simulink model "part1"  (R2020a)
settings: Solver=VariableStepAuto  StartTime=0.0  StopTime=1000  RelTol=1e-3
values from neighbouring files (symbols this model uses):
  beta_c_init = 30    [init.m]    (also in simulation1.m = 2.35619449019; simulation2.m = 3.14159265359; simulation3.m = 0; simulation4.m = 0)
  beta_c_slope = 90/1000    (= 0.09)    [init.m]    (also in simulation1.m = 0; simulation2.m = 0.00235619449019; simulation3.m = 0; simulation4.m = 0)
  eta_d = [50 0 0; 50 -50 0; 50 -50 pi/2; 0 -50 pi/2; 0 0 0]    [init.m]    (also in simulation1.m = [0 0 0; 0 0 0]; simulation2.m = [0 0 0; 0 0 0]; simulation3.m = [0 0 0; 10 10 3*pi/2]; simulation4.m = [0 0 0; 50 0 0; 50 -50 0; 50 -50 -pi/4; 0 -50 -pi/4; 0 0 0])
  Kd = eye(n)*kd    [control_law.m]
  Ki = eye(n)*ki    [control_law.m]    (also in lqr_error.m = lqr(Aa,Ba,Qa,R); lqr_integral.m = lqr(Aa,Ba,Qa,R))
  Kp = eye(n)*kp    [control_law.m]
  V_c = input    [gui.m]    (also in init.m = 0.5; simulation1.m = 0.5; simulation2.m = 0.5; simulation3.m = 0)
undefined symbols (not defined in the file or in its folder): DiscIntNeverNeededParam, Hoerner, vessel
libraries: marine_gnc x11, simulink x2, marine_hydro x1
settings Model: OrderedModelArguments=off  Creator=jonbjor  LastModifiedBy=magnushaukeland
settings DataIOCC: ReturnWorkspaceOutputs=off
settings DebuggingCC: ArithmeticOperatorsInVariantConditions=warning
settings SFSimCC: SimUseLocalCustomCode=off  CustomCodeUndefinedFunction=UseInterfaceOnly
settings RTWCC: RTWUseLocalCustomCode=off

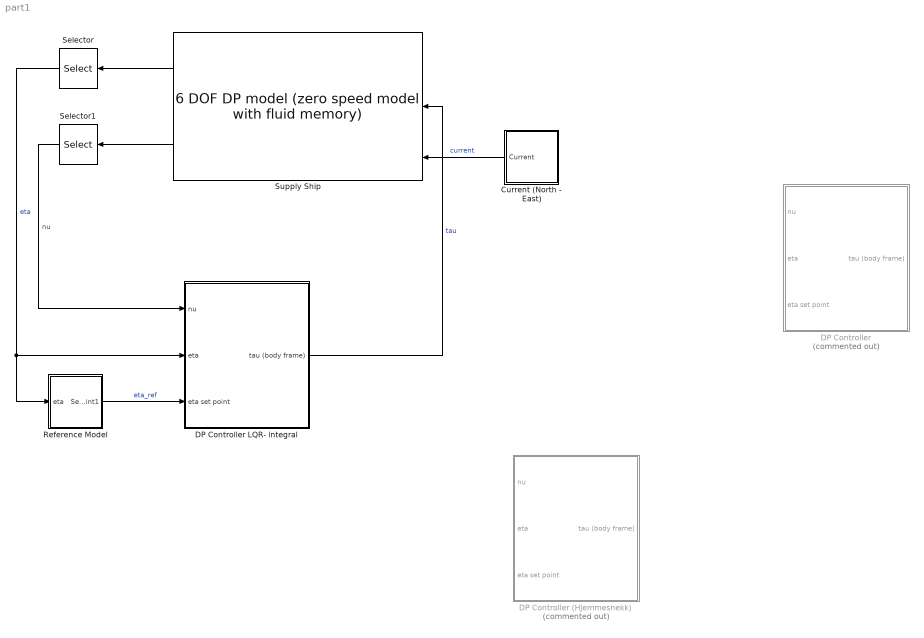
== system part1 ==
  Current (North - East) : Subsystem
  DP Controller : Subsystem  Commented=on
  DP Controller (Hjemmesnekk) : Subsystem  Commented=on
  DP Controller LQR- integral : Subsystem
  Reference Model : Subsystem
  Selector : Selector  InputPortWidth=6  IndexOptions=Index vector (dialog)  Indices=[1 2 6]  OutputSizes=1
  Selector1 : Selector  InputPortWidth=6  IndexOptions=Index vector (dialog)  Indices=[1 2 6]  OutputSizes=1
  Supply Ship : marine_hydro/Hydro Library/6 DOF DP model  (zero speed model with fluid memory)  ABC=vesselABC  rho=1025  Axc=0.9*vessel.main.T*vessel.main.B  Ayc=0.9*vessel.main.T*vessel.main.Lpp  CX=1  CY_2D=Hoerner(vessel.main.B,vessel.main.T)  Bv=vessel.Bv  mask(6 DOF zero speed model){}
      link override "Integrator1 ": InitialCondition=nu0
      link override Integrator2: InitialCondition=eta0
      settings: SourceProductName=MSS Hydro
      mask Display:
      | image('supply.jpg');
      | color('white'); port_label('output', 1, 'eta')
      | color('white'); port_label('output', 2, 'nu')
      | color('white'); port_label('input', 1, 'tau_wave')
      | color('white'); port_label('input', 2, 'tau')
      | color('white'); port_label('input', 3, 'nu_c')
  wires:
  Current (North - East)/1(Current) -> Supply Ship/3  "current"
  Supply Ship/1 -> Selector/1
  Supply Ship/2 -> Selector1/1
  Selector/1 -> DP Controller LQR- integral/2(eta), Reference Model/1(eta)  "eta"
  Reference Model/1(Set-point1) -> DP Controller LQR- integral/3(eta set point)  "eta_ref"
  Selector1/1 -> DP Controller LQR- integral/1(nu)  "nu"
  DP Controller LQR- integral/1(tau (body frame)) -> Supply Ship/2  "tau"

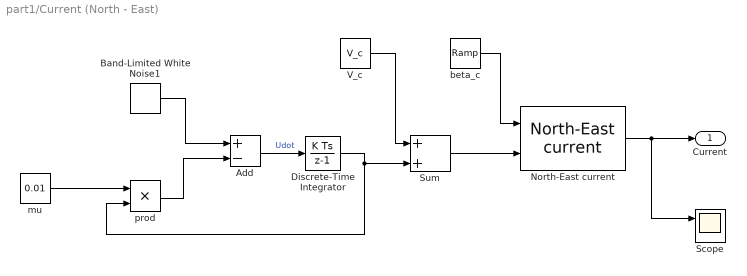
== system part1/Current (North - East) ==
  Add : Sum  Inputs=+-
  Band-Limited White Noise1 : simulink/Sources/Band-Limited White Noise  Cov=0.0005  Ts=0.1  seed=[23361]
  Discrete-Time Integrator : DiscreteIntegrator  SampleTime=-1  ICPrevOutput=DiscIntNeverNeededParam  ICPrevScaledInput=DiscIntNeverNeededParam
  North-East current : marine_gnc/Environment/Current/North-East current  SystemSampleTime=-1  Latency=0  AutoFrameSizeCalculation=off
      settings: SourceProductName=MSS GNC
  Scope : Scope  NumInputPorts=2
  Sum : Sum  Inputs=|++
  V_c : Constant  Value=V_c
  beta_c : simulink/Sources/Ramp  slope=beta_c_slope  start=0  InitialOutput=beta_c_init
  mu : Constant  Value=0.01
  prod : Product  Inputs=**
  Current : Outport  VectorParamsAs1DForOutWhenUnconnected=off
  wires:
  mu/1 -> prod/1
  prod/1 -> Add/2
  Band-Limited White Noise1/1 -> Add/1
  Add/1 -> Discrete-Time Integrator/1  "Udot"
  Discrete-Time Integrator/1 -> prod/2, Sum/2
  Sum/1 -> North-East current/2
  North-East current/1 -> Scope/1, Current/1
  beta_c/1 -> North-East current/1
  V_c/1 -> Sum/1

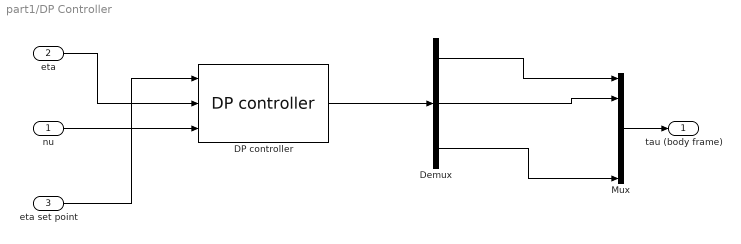
== system part1/DP Controller ==
  nu : Inport
  eta : Inport  Port=2
  eta set point : Inport  Port=3
  DP controller : marine_gnc/Control/Dynamic  Positioning /DP controller  Kp=diag([1E4 1E4 1E4])  Kd=diag([100 100 100])  Ki=diag([100 100 100])
      settings: SourceProductName=MSS GNC
  Demux : Demux  Outputs=3
  Mux : Mux  Inputs=6
  tau (body frame) : Outport  VectorParamsAs1DForOutWhenUnconnected=off
  wires:
  DP controller/1 -> Demux/1
  eta set point/1 -> DP controller/1
  nu/1 -> DP controller/3
  eta/1 -> DP controller/2
  Mux/1 -> tau (body frame)/1
  Demux/1 -> Mux/1
  Demux/2 -> Mux/2
  Demux/3 -> Mux/6

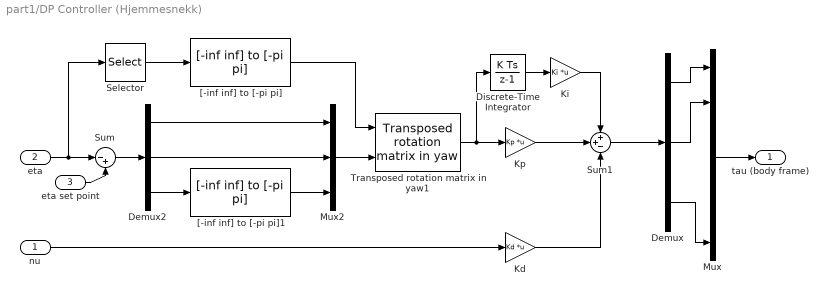
== system part1/DP Controller (Hjemmesnekk) ==
  nu : Inport
  eta : Inport  Port=2
  eta set point : Inport  Port=3
  Demux : Demux  Outputs=3
  Demux2 : Demux  Outputs=3
  Discrete-Time Integrator : DiscreteIntegrator  SampleTime=0.1  ICPrevOutput=DiscIntNeverNeededParam  ICPrevScaledInput=DiscIntNeverNeededParam
  Kd : Gain  Gain=Kd  Multiplication=Matrix(K*u)
  Ki : Gain  Gain=Ki  Multiplication=Matrix(K*u)
  Kp : Gain  Gain=Kp  Multiplication=Matrix(K*u)
  Mux : Mux  Inputs=6
  Mux2 : Mux  Inputs=3
  Selector : Selector  InputPortWidth=3  IndexOptions=Index vector (dialog)  Indices=3  OutputSizes=1
  Sum : Sum  Inputs=|-+
  Sum1 : Sum  Inputs=++-
  Transposed rotation matrix in yaw1 : marine_gnc/Models/ Kinematics/Transposed rotation  matrix in yaw
      settings: SourceProductName=MSS GNC
  "[-inf inf] to [-pi pi]" : marine_gnc/Utilities/Math Operations/[-inf inf] to [-pi pi]
      settings: SourceProductName=MSS GNC
  "[-inf inf] to [-pi pi]1" : marine_gnc/Utilities/Math Operations/[-inf inf] to [-pi pi]
      settings: SourceProductName=MSS GNC
  tau (body frame) : Outport  VectorParamsAs1DForOutWhenUnconnected=off
  wires:
  "[-inf inf] to [-pi pi]"/1 -> Transposed rotation matrix in yaw1/1
  Mux2/1 -> Transposed rotation matrix in yaw1/2
  "[-inf inf] to [-pi pi]1"/1 -> Mux2/3
  Sum/1 -> Demux2/1
  Demux2/3 -> "[-inf inf] to [-pi pi]1"/1
  Demux/3 -> Mux/6
  Demux2/2 -> Mux2/2
  eta/1 -> Sum/1, Selector/1
  Demux2/1 -> Mux2/1
  Selector/1 -> "[-inf inf] to [-pi pi]"/1
  Demux/1 -> Mux/1
  Demux/2 -> Mux/2
  Sum1/1 -> Demux/1
  Mux/1 -> tau (body frame)/1
  Ki/1 -> Sum1/1
  Kp/1 -> Sum1/2
  Transposed rotation matrix in yaw1/1 -> Discrete-Time Integrator/1, Kp/1
  Discrete-Time Integrator/1 -> Ki/1
  nu/1 -> Kd/1
  eta set point/1 -> Sum/2
  Kd/1 -> Sum1/3

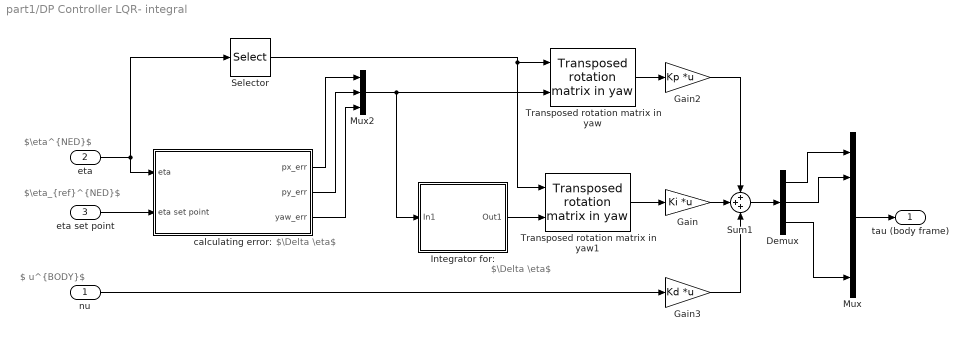
== system part1/DP Controller LQR- integral ==
  note: $\nu^{BODY}$
  note: $\eta_{ref}^{NED}$
  note: $\eta^{NED}$
  note: $\Delta \eta$
  note: $\Delta \eta$
  nu : Inport
  eta : Inport  Port=2
  eta set point : Inport  Port=3
  Demux : Demux  Outputs=3
  Gain : Gain  Gain=Ki  Multiplication=Matrix(K*u)
  Gain2 : Gain  Gain=Kp  Multiplication=Matrix(K*u)
  Gain3 : Gain  Gain=Kd  Multiplication=Matrix(K*u)
  "Integrator for: " : Subsystem
  Mux : Mux  Inputs=6
  Mux2 : Mux  Inputs=3
  Selector : Selector  InputPortWidth=3  IndexOptions=Index vector (dialog)  Indices=[3]  OutputSizes=1
  Sum1 : Sum  Inputs=+++
  Transposed rotation matrix in yaw : marine_gnc/Models/ Kinematics/Transposed rotation  matrix in yaw
      settings: SourceProductName=MSS GNC
  Transposed rotation matrix in yaw1 : marine_gnc/Models/ Kinematics/Transposed rotation  matrix in yaw
      settings: SourceProductName=MSS GNC
  "calculating error: " : Subsystem
  tau (body frame) : Outport  VectorParamsAs1DForOutWhenUnconnected=off
  wires:
  Mux/1 -> tau (body frame)/1
  Demux/2 -> Mux/2
  Demux/1 -> Mux/1
  eta set point/1 -> "calculating error: "/2(eta set point)
  Sum1/1 -> Demux/1
  nu/1 -> Gain3/1
  Gain/1 -> Sum1/2
  Gain2/1 -> Sum1/1
  Demux/3 -> Mux/6
  "calculating error: "/2(py_err) -> Mux2/2
  "calculating error: "/3(yaw_err) -> Mux2/3
  "calculating error: "/1(px_err) -> Mux2/1
  Selector/1 -> Transposed rotation matrix in yaw1/1, Transposed rotation matrix in yaw/1
  Mux2/1 -> "Integrator for: "/1(In1), Transposed rotation matrix in yaw/2
  Transposed rotation matrix in yaw/1 -> Gain2/1
  Transposed rotation matrix in yaw1/1 -> Gain/1
  eta/1 -> Selector/1, "calculating error: "/1(eta)
  "Integrator for: "/1(Out1) -> Transposed rotation matrix in yaw1/2
  Gain3/1 -> Sum1/3

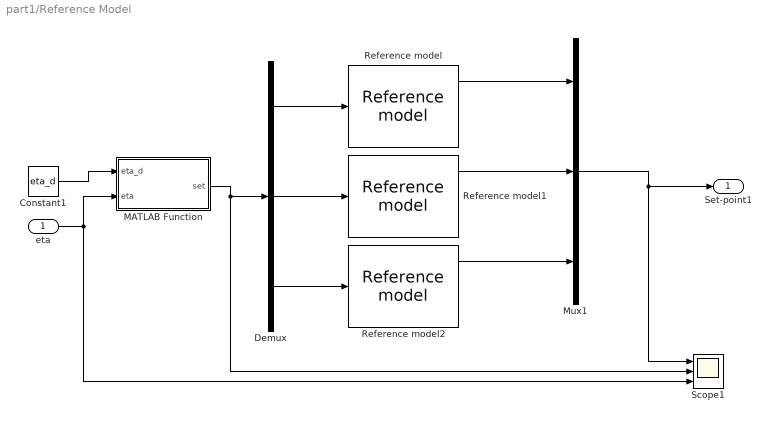
== system part1/Reference Model ==
  eta : Inport
  Constant1 : Constant  Value=eta_d
  Demux : Demux  Outputs=3
  MATLAB Function : MATLAB Function  TreatAsAtomicUnit=on
  Mux1 : Mux  Inputs=3
  Reference model : marine_gnc/Guidance/Reference model  v_max=1.0  zeta_d=1.5  w_d=0.1
      settings: SourceProductName=MSS GNC
  Reference model1 : marine_gnc/Guidance/Reference model  v_max=2  zeta_d=1.2  w_d=0.1
      settings: SourceProductName=MSS GNC
  Reference model2 : marine_gnc/Guidance/Reference model  v_max=1.0  zeta_d=1.0  w_d=0.1
      settings: SourceProductName=MSS GNC
  Scope1 : Scope  NumInputPorts=3
  Set-point1 : Outport  VectorParamsAs1DForOutWhenUnconnected=off
  wires:
  Reference model1/1 -> Mux1/2
  MATLAB Function/1(set) -> Scope1/2, Demux/1
  Demux/3 -> Reference model2/1
  Demux/2 -> Reference model1/1
  Mux1/1 -> Scope1/1, Set-point1/1
  Constant1/1 -> MATLAB Function/1(eta_d)
  Demux/1 -> Reference model/1
  Reference model/1 -> Mux1/1
  eta/1 -> Scope1/3, MATLAB Function/2(eta)
  Reference model2/1 -> Mux1/3

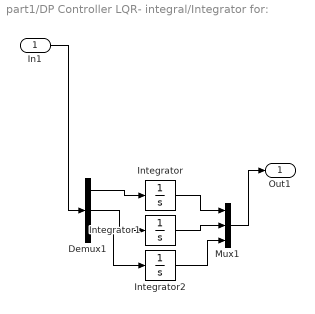
== system part1/DP Controller LQR- integral/Integrator for:  ==
  In1 : Inport
  Demux1 : Demux  Outputs=3
  Integrator : Integrator
  Integrator1 : Integrator
  Integrator2 : Integrator
  Mux1 : Mux  Inputs=3
  Out1 : Outport
  wires:
  Demux1/2 -> Integrator1/1
  Mux1/1 -> Out1/1
  Integrator2/1 -> Mux1/3
  Demux1/1 -> Integrator/1
  Integrator/1 -> Mux1/1
  In1/1 -> Demux1/1
  Demux1/3 -> Integrator2/1
  Integrator1/1 -> Mux1/2

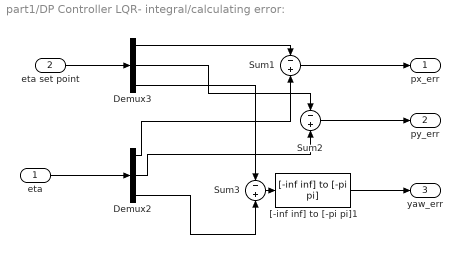
== system part1/DP Controller LQR- integral/calculating error:  ==
  eta : Inport
  eta set point : Inport  Port=2
  Demux2 : Demux  Outputs=3
  Demux3 : Demux  Outputs=3
  Sum1 : Sum  Inputs=-+
  Sum2 : Sum  Inputs=-+
  Sum3 : Sum  Inputs=-+
  "[-inf inf] to [-pi pi]1" : marine_gnc/Utilities/Math Operations/[-inf inf] to [-pi pi]
      settings: SourceProductName=MSS GNC
  px_err : Outport
  py_err : Outport  Port=2
  yaw_err : Outport  Port=3
  wires:
  eta set point/1 -> Demux3/1
  Sum3/1 -> "[-inf inf] to [-pi pi]1"/1
  Demux3/2 -> Sum2/1
  Demux3/3 -> Sum3/1
  Demux3/1 -> Sum1/1
  Demux2/2 -> Sum2/2
  Demux2/3 -> Sum3/2
  Sum1/1 -> px_err/1
  Sum2/1 -> py_err/1
  "[-inf inf] to [-pi pi]1"/1 -> yaw_err/1
  eta/1 -> Demux2/1
  Demux2/1 -> Sum1/2

== matlab function part1/Reference Model/MATLAB Function ==
  settings: updateMethod=DISCRETE
  data: eta_d input; eta input; set output
function set = cornertest(eta_d, eta)
    %corners = [50 0 0; 50 -50 0; 50 -50 pi/4; 0 -50 pi/4; 0 0 0];
    
    persistent idx
    if isempty(idx)
        idx = 1;
    end
    
    pos_margin = 0.5;
    angle_margin = 0.05;
    
    if( (abs(eta(1)-eta_d(idx,1)) < pos_margin) && ...
        (abs(eta(2)-eta_d(idx,2)) < pos_margin) && ...
        (abs(eta(3)-eta_d(idx,3)) < angle_margin) )
        %disp("SWITCHING");
        %disp(idx + 1);
        if (idx<size(eta_d,1))
            idx = idx + 1;
        end
    end
    set = eta_d(idx, :);
    disp(set)
end
